simulink model "RTA_Controller"  (R2015a)
settings: Solver=FixedStepDiscrete  StartTime=0.0  StopTime=100  FixedStep=delta_t  RelTol=1e-3
settings Model: Creator=Kerianne  LastModifiedBy=Kerianne
settings DataIOCC: SaveFormat=Structure
settings OptimizationCC: InlineParams=on  ExpressionDepthLimit=2147483647
settings DebuggingCC: UnderspecifiedInitializationDetection=Classic  MergeDetectMultiDrivingBlocksExec=none  SolverPrmCheckMsg=warning  StateNameClashWarn=warning

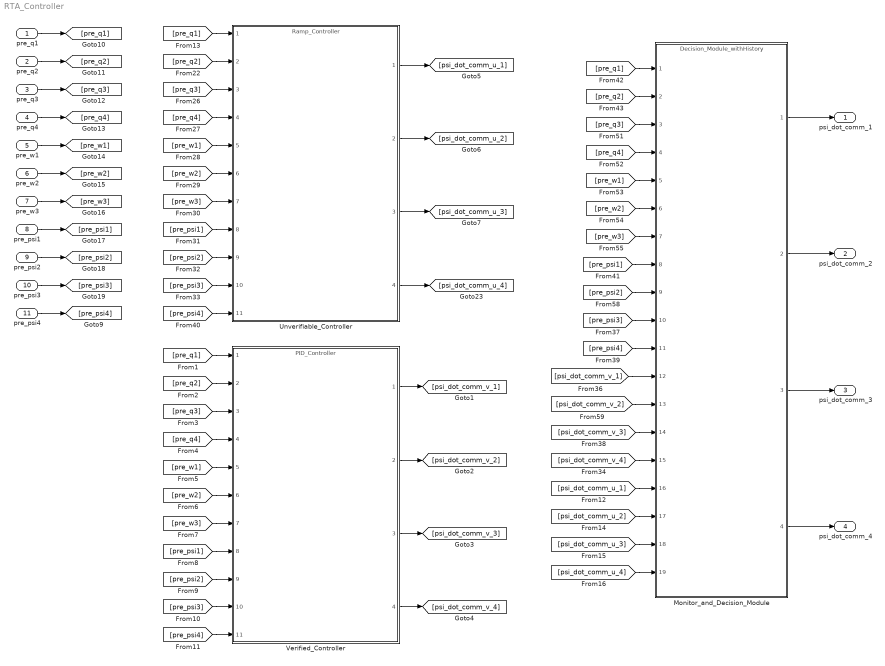
== system RTA_Controller ==
  pre_q1 : Inport
  pre_q2 : Inport  Port=2
  pre_q3 : Inport  Port=3
  pre_q4 : Inport  Port=4
  pre_w1 : Inport  Port=5
  pre_w2 : Inport  Port=6
  pre_w3 : Inport  Port=7
  pre_psi1 : Inport  Port=8
  pre_psi2 : Inport  Port=9
  pre_psi3 : Inport  Port=10
  pre_psi4 : Inport  Port=11
  Monitor_and_Decision_Module : ModelReference  ModelNameDialog=Decision_Module_withHistory.slx  SimulationMode=Normal  ModelReferenceVersion=1.60  CopyOfModelName=Decision_Module_withHistory.slx  DefaultDataLogging=on
  Unverifiable_Controller : ModelReference  ModelNameDialog=Ramp_Controller.slx  SimulationMode=Normal  ModelReferenceVersion=1.18  CopyOfModelName=Ramp_Controller.slx  DefaultDataLogging=on
  Verified_Controller : ModelReference  ModelNameDialog=PID_Controller.slx  SimulationMode=Normal  ModelReferenceVersion=1.22  CopyOfModelName=PID_Controller.slx  DefaultDataLogging=on
  psi_dot_comm_1 : Outport
  psi_dot_comm_2 : Outport  Port=2
  psi_dot_comm_3 : Outport  Port=3
  psi_dot_comm_4 : Outport  Port=4
  wires:
  [pre_q1] -> Unverifiable_Controller/1
  [pre_q2] -> Unverifiable_Controller/2
  [pre_q3] -> Unverifiable_Controller/3
  [pre_q4] -> Unverifiable_Controller/4
  [pre_w1] -> Unverifiable_Controller/5
  [pre_w2] -> Unverifiable_Controller/6
  [pre_w3] -> Unverifiable_Controller/7
  [pre_psi1] -> Unverifiable_Controller/8
  [pre_psi2] -> Unverifiable_Controller/9
  [pre_psi3] -> Unverifiable_Controller/10
  pre_q1/1 -> [pre_q1]
  pre_q2/1 -> [pre_q2]
  pre_q3/1 -> [pre_q3]
  pre_q4/1 -> [pre_q4]
  pre_w1/1 -> [pre_w1]
  pre_w2/1 -> [pre_w2]
  pre_w3/1 -> [pre_w3]
  pre_psi1/1 -> [pre_psi1]
  pre_psi2/1 -> [pre_psi2]
  pre_psi3/1 -> [pre_psi3]
  pre_psi4/1 -> [pre_psi4]
  [pre_psi4] -> Unverifiable_Controller/11
  Monitor_and_Decision_Module/1 -> psi_dot_comm_1/1
  Monitor_and_Decision_Module/2 -> psi_dot_comm_2/1
  Monitor_and_Decision_Module/3 -> psi_dot_comm_3/1
  [pre_psi1] -> Monitor_and_Decision_Module/8
  [pre_psi2] -> Monitor_and_Decision_Module/9
  [pre_psi3] -> Monitor_and_Decision_Module/10
  [pre_w3] -> Monitor_and_Decision_Module/7
  [pre_w2] -> Monitor_and_Decision_Module/6
  [pre_w1] -> Monitor_and_Decision_Module/5
  [pre_q4] -> Monitor_and_Decision_Module/4
  [pre_q3] -> Monitor_and_Decision_Module/3
  [pre_q2] -> Monitor_and_Decision_Module/2
  [pre_q1] -> Monitor_and_Decision_Module/1
  Monitor_and_Decision_Module/4 -> psi_dot_comm_4/1
  [pre_psi4] -> Monitor_and_Decision_Module/11
  [psi_dot_comm_v_1] -> Monitor_and_Decision_Module/12
  [psi_dot_comm_v_2] -> Monitor_and_Decision_Module/13
  [psi_dot_comm_v_3] -> Monitor_and_Decision_Module/14
  [psi_dot_comm_v_4] -> Monitor_and_Decision_Module/15
  [pre_q1] -> Verified_Controller/1
  [pre_q2] -> Verified_Controller/2
  [pre_q3] -> Verified_Controller/3
  [pre_q4] -> Verified_Controller/4
  [pre_w1] -> Verified_Controller/5
  [pre_w2] -> Verified_Controller/6
  [pre_w3] -> Verified_Controller/7
  [pre_psi1] -> Verified_Controller/8
  [pre_psi2] -> Verified_Controller/9
  [pre_psi3] -> Verified_Controller/10
  [pre_psi4] -> Verified_Controller/11
  [psi_dot_comm_u_1] -> Monitor_and_Decision_Module/16
  [psi_dot_comm_u_2] -> Monitor_and_Decision_Module/17
  [psi_dot_comm_u_3] -> Monitor_and_Decision_Module/18
  [psi_dot_comm_u_4] -> Monitor_and_Decision_Module/19
  Unverifiable_Controller/1 -> [psi_dot_comm_u_1]
  Unverifiable_Controller/2 -> [psi_dot_comm_u_2]
  Unverifiable_Controller/3 -> [psi_dot_comm_u_3]
  Unverifiable_Controller/4 -> [psi_dot_comm_u_4]
  Verified_Controller/1 -> [psi_dot_comm_v_1]
  Verified_Controller/2 -> [psi_dot_comm_v_2]
  Verified_Controller/3 -> [psi_dot_comm_v_3]
  Verified_Controller/4 -> [psi_dot_comm_v_4]
